simulink model "lab5"  (R2023a)
settings: Solver=VariableStepAuto  StartTime=0.0  StopTime=inf  RelTol=1e-3
undefined symbols (not defined in the file): CR, LF
libraries: instrumentseriallib x2
settings Model: Creator=vasil  LastModifiedBy=vasil

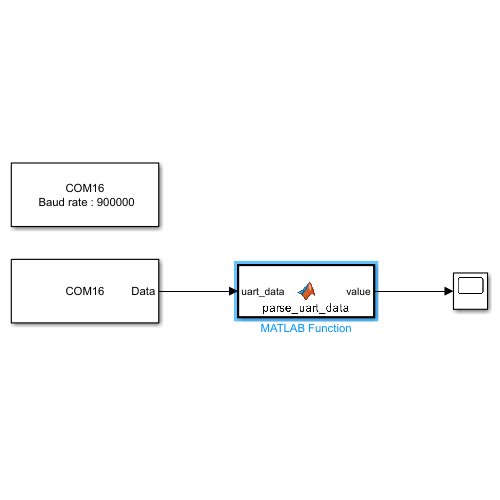
[thumbnail: Simulink's stored preview of the top-level diagram]
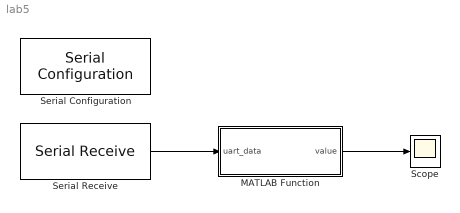
== system lab5 ==
  MATLAB Function : MATLAB Function  TreatAsAtomicUnit=on
  Scope : Scope
  Serial Configuration : instrumentseriallib/Serial Configuration  Priority=-200000  PortSel=COM16  Port=COM16  ComPort=COM16  BaudRate=900000  DataBits=8  Parity=none  StopBits=1  ByteOrder=little-endian  FlowControl=none  Timeout=10  SimulateUsing=Interpreted execution  BlockInModel=on  aMode=1
  Serial Receive : instrumentseriallib/Serial Receive  Priority=1  PortSel=COM16  Port=COM16  ComPort=COM16  DataType=uint8  SaveDataType=uint8  ToggleHeader=off  Header=['v=']  ToggleTerminator=off  Terminator=CR/LF ('\r\n')  CustomTerminator=['\0', '\r', '\n']  InputFormat=Column major  ToggleDataSize=on  DataSize=[32 1]  EnableBlockingMode=on  ActionDataUnavailable=Error  ActionWhenDataUnavailable=Error  CustomValue=0  SampleTime=1/1000  SimulateUsing=Interpreted execution  BlockInModel=on  aMode=1
  wires:
  Serial Receive/1 -> MATLAB Function/1(uart_data)
  MATLAB Function/1(value) -> Scope/1

== matlab function lab5/MATLAB Function ==
  data: uart_data input; value output
function value = parse_uart_data(uart_data)
    persistent buffer
    if isempty(buffer)
        buffer = '';
    end
    
    % Преобразуем uint8 данные в строку и добавляем к буферу
    str = char(uart_data');
    buffer = strcat(buffer, str); % накопление данных в буфере
    
    % Поиск начала и конца строки
    start_pos = strfind(buffer, 'v='); % позиция начала данных
    end_pos = strfind(buffer, '\r\n'); % позиция конца данных
    
    if ~isempty(start_pos) && ~isempty(end_pos) && end_pos(1) > start_pos(1)
        % Извлечение подстроки между 'v=' и '\r\n'
        value_str = buffer(start_pos(1) + 2 : end_pos(1) - 1); % извлечение значения после 'v='
        
        % Конвертация извлеченной строки в число
        value = str2double(value_str);
        
        % Очистка буфера до конца обработанной строки
        buffer = buffer(end_pos(1) + 2:end); % оставляем остаток данных, если он есть
    else
        value = NaN; % пока не получены все данные
    end
end
